simulink model "simulink_observador"  (R2014b)
settings: Solver=ode45  StartTime=0.0  StopTime=25  MaxStep=0.001  RelTol=1e-3
values from neighbouring files (symbols this model uses):
  A = [0 1 0; 0 -b/J K/J; 0 -K/L R/L]    [control_pos.m]    (also in identificacio.mat = [-865.972596766  300.341767754; -74.9918164222  0.0087686494; observador.m = [-b/J K/J; -K/L R/L]; plot_iden.m = [-b/J K/J; -K/L R/L])
  B = [0; 0; 1/L]    [control_pos.m]    (also in identificacio.mat = [0 74.7570280889]; observador.m = [0; 1/L]; plot_iden.m = [0; 1/L])
  C = [1,0,0]    [control_pos.m]    (also in identificacio.mat = [1 0]; observador.m = [1,0]; plot_iden.m = [1,0])
  D = 0    [control_pos.m]    (also in identificacio.mat; observador.m; plot_iden.m)
  K_dis = acker(phi,gam,P_dis)    [control_pos.m]    (also in observador.m)
  L = 0.013376668730204    (= 0.0133766687302)    [control_pos.m]    (also in identificacio.mat; observador.m)
  Nu = N(4)    [control_pos.m]    (also in observador.m = N(3))
  Nx = N(1:3)    [control_pos.m]    (also in observador.m = N(1:2))
undefined symbols (not defined in the file or in its folder): gam, phi
settings Model: Creator=student  LastModifiedBy=lluis
settings DataIOCC: SignalLoggingSaveFormat=ModelDataLogs
settings OptimizationCC: ExpressionDepthLimit=2147483647
settings DebuggingCC: UnderspecifiedInitializationDetection=Classic  MergeDetectMultiDrivingBlocksExec=none  FcnCallInpInsideContextMsg=EnableAllAsWarning  StateNameClashWarn=warning
settings GRTTargetCC: CombineOutputUpdateFcns=off  GRTInterface=on

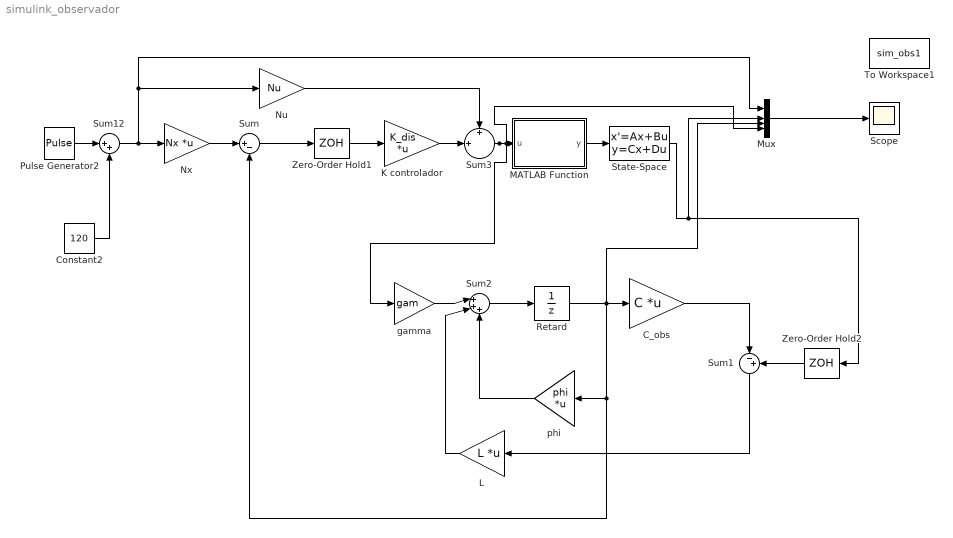
== system simulink_observador ==
  C_obs : Gain  Gain=C  Multiplication=Matrix(K*u)
  Constant2 : Constant  Value=120
  K controlador : Gain  Gain=K_dis  Multiplication=Matrix(K*u)
  L : Gain  Gain=L  Multiplication=Matrix(K*u)
  MATLAB Function : MATLAB Function  TreatAsAtomicUnit=on
  Mux : Mux  Inputs=5
  Nu : Gain  Gain=Nu
  Nx : Gain  Gain=Nx  Multiplication=Matrix(K*u)
  Pulse Generator2 : DiscretePulseGenerator  PulseType=Time based  Amplitude=40  Period=5  PulseWidth=50
  Retard : UnitDelay  SampleTime=-1
  Scope : Scope
  State-Space : StateSpace  A=A  B=B  C=C  D=D  X0=[1;1]
  Sum : Sum  Inputs=|+-
  Sum1 : Sum  Inputs=|-+
  Sum12 : Sum  Inputs=|++
  Sum2 : Sum  Inputs=|+++
  Sum3 : Sum  Inputs=+|+||
  To Workspace1 : ToWorkspace  VariableName=sim_obs1  SaveFormat=Timeseries  SampleTime=-1
  Zero-Order Hold1 : ZeroOrderHold  SampleTime=5E-2
  Zero-Order Hold2 : ZeroOrderHold  SampleTime=5E-2
  gamma : Gain  Gain=gam
  phi : Gain  Gain=phi  Multiplication=Matrix(K*u)
  wires:
  Sum/1 -> Zero-Order Hold1/1
  Nx/1 -> Sum/1
  Zero-Order Hold1/1 -> K controlador/1
  Sum1/1 -> L/1
  gamma/1 -> Sum2/1
  L/1 -> Sum2/2
  Retard/1 -> C_obs/1, phi/1, Sum/2, Mux/4
  Sum2/1 -> Retard/1
  phi/1 -> Sum2/3
  State-Space/1 -> Zero-Order Hold2/1, Mux/3
  C_obs/1 -> Sum1/1
  Zero-Order Hold2/1 -> Sum1/2
  Sum12/1 -> Nu/1, Mux/1, Nx/1
  Pulse Generator2/1 -> Sum12/1
  Constant2/1 -> Sum12/2
  K controlador/1 -> Sum3/2
  Nu/1 -> Sum3/1
  Mux/1 -> Scope/1
  Sum3/1 -> Mux/5, gamma/1, MATLAB Function/1(u)
  MATLAB Function/1(y) -> State-Space/1

== matlab function simulink_observador/MATLAB Function ==
  data: u input; y output
function y = fcn(u)
%#codegen
y = 0.0004087630826036687*u^3 - 0.141361790772926*u^2 + 17.097698790218242*u - 620.9671400241792;
end
